simulink model "schema"  (R2018b)
settings: Solver=ode1  StartTime=current_tmin  StopTime=current_tmax  FixedStep=h_step  RelTol=1e-3
values from neighbouring files (symbols this model uses):
  current_tmin = 0    [start_simulation.m]
  dist_left = f_pos(1) + ax_pos(1)    [compute_screen_parameters.m]    (also in read_cursor_input.m = in(5); start_simulation.m = nan)
  dist_lower = f_pos(2) + ax_pos(2)    [compute_screen_parameters.m]    (also in read_cursor_input.m = in(6); start_simulation.m = nan)
  dist_right = screen_width - dist_left - ax_pos(3)    [compute_screen_parameters.m]    (also in read_cursor_input.m = in(7); start_simulation.m = nan)
  dist_upper = screen_height - dist_lower - ax_pos(4)    [compute_screen_parameters.m]    (also in read_cursor_input.m = in(8); start_simulation.m = nan)
  h_step = 0.01    [prepare_simulation.m]    (also in start_simulation.m = sim_struct.h_step)
  l1 = in(2)    [invert_J.m]    (also in plot_robot_position.m = in(3); read_cursor_input.m = in(1); start_simulation.m = sim_struct.l1)
  l2 = in(3)    [invert_J.m]    (also in plot_robot_position.m = in(4); read_cursor_input.m = in(2); start_simulation.m = sim_struct.l2)
  plot_mode = 2    [plot_mode_str2int.m]    (also in plot_robot_position.m = in(5); prepare_simulation.m = plot_mode_str2int(plot_mode); start_simulation.m = sim_struct.plot_mode_num)
  q1iws = 0    [start_simulation.m]
  q2iws = 0;  xstar{n} = [0 0 0]; xstardot{n} = [0 0 0]    [start_simulation.m]
  screen_height = screen_size(4)    [compute_screen_parameters.m]    (also in read_cursor_input.m = in(4); start_simulation.m = nan)
  screen_width = screen_size(3)    [compute_screen_parameters.m]    (also in read_cursor_input.m = in(3); start_simulation.m = nan)
  sw = in(7)    [invert_J.m]    (also in plot_robot_position.m = in(11); prepare_offline_given.m = 1; prepare_offline_manual.m = 2; prepare_simulation.m = -1)
  vmax = in(8)    [invert_J.m]    (also in start_simulation.m = sim_struct.vmax)
libraries: simulink x1
settings Model: SimulationMode=accelerator  Creator=HEW15BS514NL  LastModifiedBy=HEW15BS514NL
settings DataIOCC: SaveState=on
settings OptimizationCC: EfficientMapNaN2IntZero=off
settings HardwareCC: TargetBitPerPointer=64  TargetBitPerSizeT=64  TargetBitPerPtrDiffT=64  TargetLongLongMode=on  TargetIntDivRoundTo=Zero  TargetEndianess=LittleEndian  TargetWordSize=64  TargetHWDeviceType=MATLAB Host  ProdEqTarget=off
settings CodeAppCC: MaxIdLength=128
settings GRTTargetCC: TargetLangStandard=C89/C90 (ANSI)  CombineOutputUpdateFcns=off  GRTInterface=on

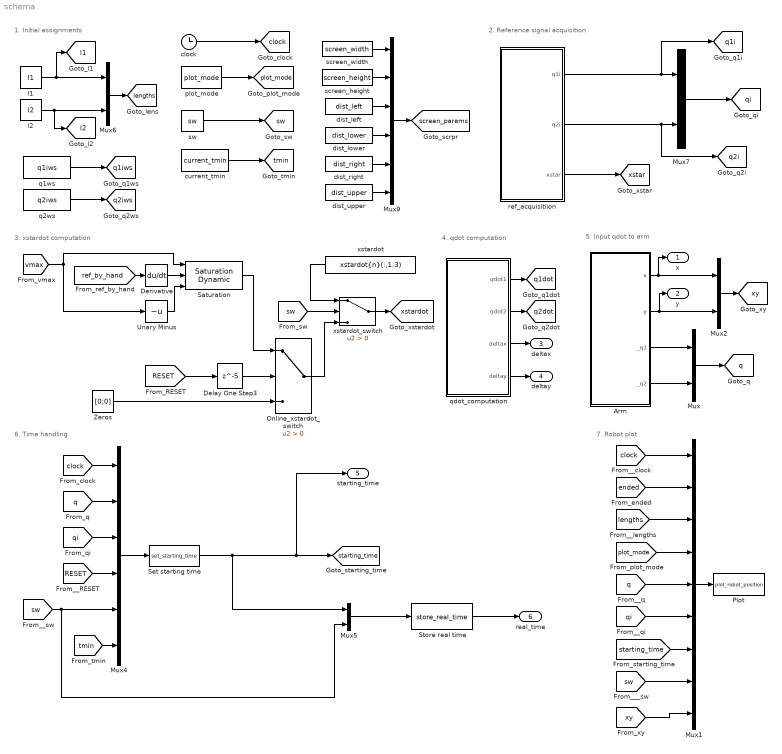
== system schema ==
  note: 4. qdot computation
  note: 3. xstardot computation
  note: 2. Reference signal acquisition
  note: 5. Input qdot to arm
  note: 7. Robot plot
  note: 6. Time handling
  note: 1. Initial assignments
  Arm : Subsystem
  Delay One Step3 : Delay  DelayLength=5
  Derivative : Derivative
  Mux{,2,5..7} (5 alike) : Mux  Inputs=2
  Mux1 : Mux  Inputs=9
  Mux4 : Mux  Inputs=6
  Mux9 : Mux  Inputs=6
  Online_xstardot_switch : Switch  Criteria=u2 > Threshold
  Plot : MATLABFcn  MATLABFcn=plot_robot_position  OutputDimensions=0  Output1D=off
  Saturation : simulink/Discontinuities/Saturation Dynamic  OutMin=[]  OutMax=[]  OutDataTypeStr=Inherit: Same as second input  OutDataType=fixdt(1, 16)  OutScaling=2^-10  DoSatur=off
  Set starting time : MATLABFcn  MATLABFcn=set_starting_time  OutputDimensions=1  OutputSignalType=real
  Store real time : MATLABFcn  MATLABFcn=store_real_time  OutputDimensions=1
  Unary Minus : UnaryMinus
  Zeros : Constant  Value=[0;0]
  clock : Clock
  current_tmin : Constant  Value=current_tmin
  dist_left : Constant  Value=dist_left
  dist_lower : Constant  Value=dist_lower
  dist_right : Constant  Value=dist_right
  dist_upper : Constant  Value=dist_upper
  l1 : Constant  Value=l1
  l2 : Constant  Value=l2
  plot_mode : Constant  Value=plot_mode
  q1ws : Constant  Value=q1iws  SampleTime=-1
  q2ws : Constant  Value=q2iws  SampleTime=-1
  qdot_computation : Subsystem
  ref_acquisitiion : Subsystem
  screen_height : Constant  Value=screen_height
  screen_width : Constant  Value=screen_width
  sw : Constant  Value=sw
  xstardot : FromWorkspace  VariableName=xstardot{n}(:,1:3)  SampleTime=0
  xstardot_switch : Switch  Criteria=u2 > Threshold
  x : Outport
  y : Outport  Port=2
  deltax : Outport  Port=3
  deltay : Outport  Port=4
  starting_time : Outport  Port=5
  real_time : Outport  Port=6
  tag scope: clock=global, l1=global, l2=global, lengths=global, plot_mode=global, q1dot=global, q1i=global, q1iws=global, q2dot=global, q2i=global, q2iws=global, q=global, qi=global, screen_params=global, starting_time=global, sw=global, tmin=global, xstar=global, xstardot=global, xy=global
  wires:
  Mux1/1 -> Plot/1
  xstardot_switch/1 -> [xstardot]
  Zeros/1 -> Online_xstardot_switch/3
  Online_xstardot_switch/1 -> xstardot_switch/3
  [RESET] -> Delay One Step3/1
  [sw] -> xstardot_switch/2
  [ref_by_hand] -> Derivative/1
  Delay One Step3/1 -> Online_xstardot_switch/2
  xstardot/1 -> xstardot_switch/1
  Mux4/1 -> Set starting time/1
  Saturation/1 -> Online_xstardot_switch/1
  Unary Minus/1 -> Saturation/3
  [clock] -> Mux1/1
  [ended] -> Mux1/2
  [lengths] -> Mux1/3
  [xy] -> Mux1/9
  [sw] -> Mux1/8
  [starting_time] -> Mux1/7
  [plot_mode] -> Mux1/4
  [q] -> Mux1/5
  [qi] -> Mux1/6
  [tmin] -> Mux4/6
  [clock] -> Mux4/1
  [RESET] -> Mux4/4
  [q] -> Mux4/2
  [qi] -> Mux4/3
  [sw] -> Mux4/5, Mux5/2
  Store real time/1 -> real_time/1
  Mux5/1 -> Store real time/1
  Set starting time/1 -> starting_time/1, [starting_time], Mux5/1
  current_tmin/1 -> [tmin]
  clock/1 -> [clock]
  plot_mode/1 -> [plot_mode]
  l2/1 -> [l2], Mux6/2
  Mux6/1 -> [lengths]
  l1/1 -> Mux6/1, [l1]
  sw/1 -> [sw]
  dist_left/1 -> Mux9/3
  Mux9/1 -> [screen_params]
  screen_width/1 -> Mux9/1
  dist_right/1 -> Mux9/5
  screen_height/1 -> Mux9/2
  dist_upper/1 -> Mux9/6
  dist_lower/1 -> Mux9/4
  Mux7/1 -> [qi]
  ref_acquisitiion/1("q1i ") -> Mux7/1, [q1i]
  ref_acquisitiion/2(q2i) -> [q2i], Mux7/2
  ref_acquisitiion/3("xstar ") -> [xstar]
  qdot_computation/1(qdot1) -> [q1dot]
  qdot_computation/2(qdot2) -> [q2dot]
  qdot_computation/3(deltax) -> deltax/1
  qdot_computation/4(deltay) -> deltay/1
  Arm/4(_q2) -> Mux/2
  Mux/1 -> [q]
  Arm/2(y) -> Mux2/2, y/1
  Arm/1(x) -> x/1, Mux2/1
  Mux2/1 -> [xy]
  Arm/3("_q1 ") -> Mux/1
  q1ws/1 -> [q1iws]
  q2ws/1 -> [q2iws]
  Derivative/1 -> Saturation/2
  [vmax] -> Unary Minus/1, Saturation/1

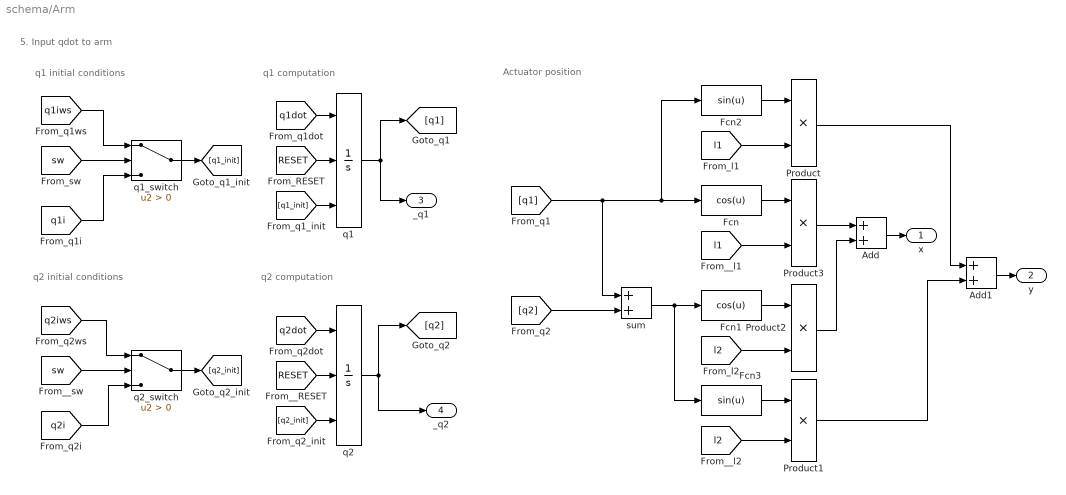
== system schema/Arm ==
  note: 5. Input qdot to arm
  note: Actuator position
  note: q2 computation
  note: q1 computation
  note: q2 initial conditions
  note: q1 initial conditions
  Add : Sum
  Add1 : Sum
  Fcn : Fcn  Expr=cos(u)
  Fcn1 : Fcn  Expr=cos(u)
  Fcn2 : Fcn  Expr=sin(u)
  Fcn3 : Fcn  Expr=sin(u)
  Product{,1..3} (4 alike) : Product
  q1 : Integrator  ExternalReset=either  InitialConditionSource=external
  q1_switch : Switch  Criteria=u2 > Threshold
      settings: LockScale=on
  q2 : Integrator  ExternalReset=either  InitialConditionSource=external  InitialCondition=0.5
  q2_switch : Switch  Criteria=u2 > Threshold
      settings: LockScale=on
  sum : Sum
  x : Outport
  y : Outport  Port=2
  "_q1 " : Outport  Port=3
  _q2 : Outport  Port=4
  wires:
  [q2dot] -> q2/1
  [q1dot] -> q1/1
  Add1/1 -> y/1
  sum/1 -> Fcn3/1, Fcn1/1
  [q1iws] -> q1_switch/1
  [sw] -> q1_switch/2
  [q1i] -> q1_switch/3
  [q2i] -> q2_switch/3
  [q2iws] -> q2_switch/1
  [sw] -> q2_switch/2
  [RESET] -> q1/2
  q1_switch/1 -> [q1_init]
  [q1_init] -> q1/3
  q2_switch/1 -> [q2_init]
  [q2_init] -> q2/3
  [RESET] -> q2/2
  [q1] -> sum/1, Fcn2/1, Fcn/1
  q1/1 -> [q1], "_q1 "/1
  q2/1 -> [q2], _q2/1
  Product/1 -> Add1/1
  Fcn3/1 -> Product1/1
  Product1/1 -> Add1/2
  [l2] -> Product1/2
  Fcn1/1 -> Product2/1
  [l2] -> Product2/2
  Product2/1 -> Add/2
  Fcn/1 -> Product3/1
  Product3/1 -> Add/1
  [l1] -> Product3/2
  Fcn2/1 -> Product/1
  [l1] -> Product/2
  [q2] -> sum/2
  Add/1 -> x/1

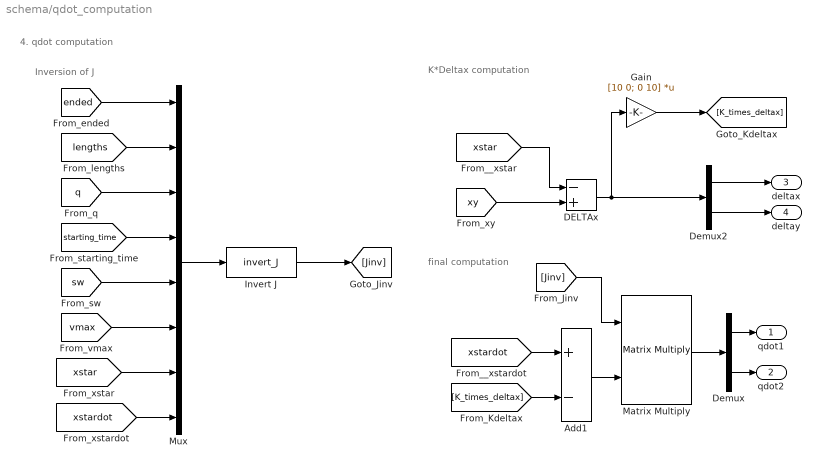
== system schema/qdot_computation ==
  note: 4. qdot computation
  note: final computation
  note: K*Deltax computation
  note: Inversion of J
  Add1 : Sum  Inputs=+-
  DELTAx : Sum  Inputs=-+
  Demux : Demux  Outputs=2
  Demux2 : Demux  Outputs=2
  Gain : Gain  Gain=[10 0; 0 10]  Multiplication=Matrix(K*u)
  Invert J : MATLABFcn  MATLABFcn=invert_J  OutputDimensions=[2;2]  Output1D=off
  Matrix Multiply : Product  Multiplication=Matrix(*)
  Mux : Mux  Inputs=8
  qdot1 : Outport
  qdot2 : Outport  Port=2
  deltax : Outport  Port=3
  deltay : Outport  Port=4
  wires:
  [xstar] -> DELTAx/1
  [xy] -> DELTAx/2
  Add1/1 -> Matrix Multiply/2
  Matrix Multiply/1 -> Demux/1
  [xstardot] -> Add1/1
  [Jinv] -> Matrix Multiply/1
  Invert J/1 -> [Jinv]
  Gain/1 -> [K_times_deltax]
  [K_times_deltax] -> Add1/2
  Mux/1 -> Invert J/1
  Demux2/1 -> deltax/1
  DELTAx/1 -> Gain/1, Demux2/1
  Demux2/2 -> deltay/1
  [ended] -> Mux/1
  [lengths] -> Mux/2
  [q] -> Mux/3
  [starting_time] -> Mux/4
  [sw] -> Mux/5
  [vmax] -> Mux/6
  [xstardot] -> Mux/8
  [xstar] -> Mux/7
  Demux/1 -> qdot1/1
  Demux/2 -> qdot2/1

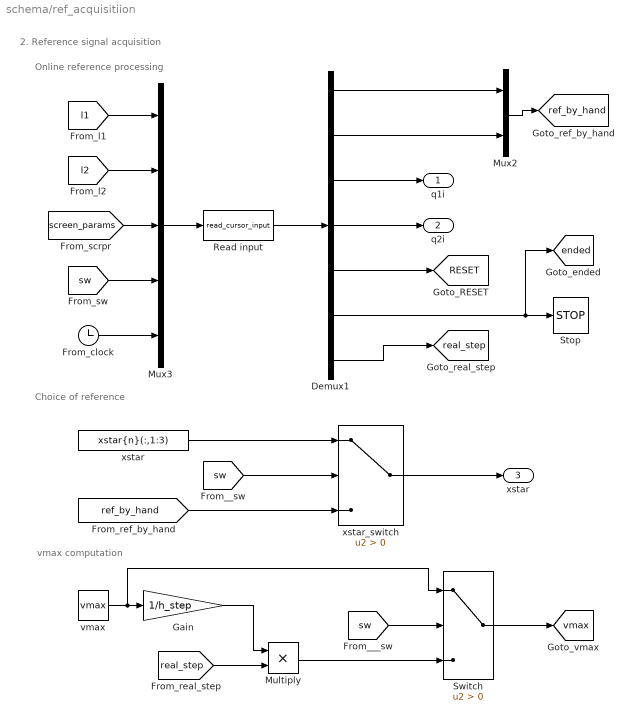
== system schema/ref_acquisitiion ==
  note: vmax computation
  note: 2. Reference signal acquisition
  note: Choice of reference
  note: Online reference processing
  Demux1 : Demux  Outputs=7
  From_clock : Clock
  Gain : Gain  Gain=1/h_step
  Multiply : Product
  Mux2 : Mux  Inputs=2
  Mux3 : Mux  Inputs=5
  Read input : MATLABFcn  MATLABFcn=read_cursor_input  OutputDimensions=[7;1]  Output1D=off
  Stop : Stop
  Switch : Switch  Criteria=u2 > Threshold
  vmax : Constant  Value=vmax
  xstar : FromWorkspace  VariableName=xstar{n}(:,1:3)  SampleTime=0
  xstar_switch : Switch  Criteria=u2 > Threshold
  "q1i " : Outport
  q2i : Outport  Port=2
  "xstar " : Outport  Port=3
  tag scope: RESET=global, ended=global, real_step=global, ref_by_hand=global, vmax=global
  wires:
  Demux1/6 -> [ended], Stop/1
  Mux3/1 -> Read input/1
  xstar/1 -> xstar_switch/1
  Demux1/3 -> "q1i "/1
  Demux1/4 -> q2i/1
  [ref_by_hand] -> xstar_switch/3
  [screen_params] -> Mux3/3
  From_clock/1 -> Mux3/5
  Demux1/1 -> Mux2/1
  [sw] -> Mux3/4
  [l2] -> Mux3/2
  Read input/1 -> Demux1/1
  [sw] -> xstar_switch/2
  Demux1/5 -> [RESET]
  Mux2/1 -> [ref_by_hand]
  xstar_switch/1 -> "xstar "/1
  [l1] -> Mux3/1
  Demux1/2 -> Mux2/2
  Demux1/7 -> [real_step]
  Gain/1 -> Multiply/1
  vmax/1 -> Switch/1, Gain/1
  Switch/1 -> [vmax]
  Multiply/1 -> Switch/3
  [sw] -> Switch/2
  [real_step] -> Multiply/2
